simulink model "autopilot"  (R2016a)
settings: Solver=VariableStepAuto  StartTime=0.0  StopTime=inf  FixedStep=0.05  RelTol=1e-3
libraries: xpcutilitieslib x2, xpcobsoletelib x2, instrumentlib x2
settings Model: Creator=IEE12  LastModifiedBy=Marcelo
settings DataIOCC: LimitDataPoints=on  SaveFormat=Array
settings DebuggingCC: UnderspecifiedInitializationDetection=Classic  MergeDetectMultiDrivingBlocksExec=none  SolverPrmCheckMsg=warning  StateNameClashWarn=warning
settings HardwareCC: ProdBitPerPointer=32  ProdLargestAtomicFloat=None  ProdIntDivRoundTo=Undefined  ProdEndianess=Unspecified  ProdWordSize=32  ProdHWDeviceType=32-bit Generic
settings ModelReferenceCC: PropagateSignalLabelsOutOfModel=off
settings ConfigComp: CovModelRefEnable=Off

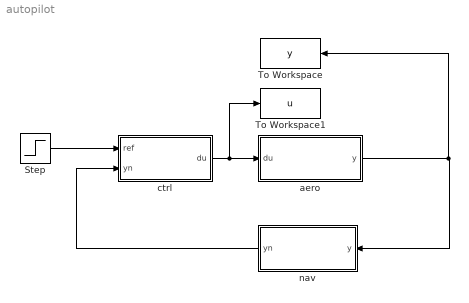
== system autopilot ==
  Step : Step  After=5  SampleTime=0
  To Workspace : ToWorkspace  VariableName=y  SaveFormat=Timeseries  SampleTime=-1
  To Workspace1 : ToWorkspace  VariableName=u  SaveFormat=Timeseries  SampleTime=-1
  aero : Subsystem
  ctrl : Subsystem
  nav : Subsystem
  wires:
  nav/1(yn) -> ctrl/2(yn)
  Step/1 -> ctrl/1(ref)
  ctrl/1(du) -> To Workspace1/1, aero/1(du)
  aero/1("y ") -> To Workspace/1, nav/1(y)

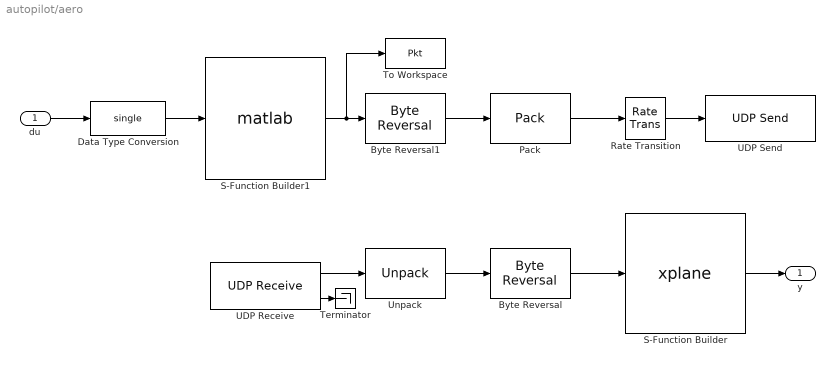
== system autopilot/aero ==
  du : Inport
  Byte Reversal : xpcutilitieslib/Byte Reversal   numInp=1
  Byte Reversal1 : xpcutilitieslib/Byte Reversal   numInp=1
  Data Type Conversion : DataTypeConversion  OutDataTypeStr=single
  Pack : xpcobsoletelib/Utilities/Pack   datatypes={'uint8'}  byteAlign=1
  Rate Transition : RateTransition  OutPortSampleTime=0.05
  S-Function Builder : S-Function  InitFcn=try, set_param(gcb,'FunctionName','xplane'), end  FunctionName=xplane  SFunctionModules=xplane_wrapper  SFunctionDeploymentMode=off  EnableBusSupport=off  mask(S-Function Builder){}
      mask help: Simulink:masks:SFunctionBuilder_MD
      mask init:
      | val = [[.9  0.75 0.75 1 1 .9 .9 1]',[1 1 0.75 0.75 .9 .9 1 .9]'];try , sys = get_param(gcb,'SfunBuilderFcnName');if isempty(sys), sys = get_param(gcb,'FunctionName'); end,catch, sys = get_param(gcb,'FunctionName'); end
      settings: CopyFcn=set_param(gcbh,'LinkStatus','none')  PreSaveFcn=try, set_param(gcb,'FunctionName','xplane'), end  OpenFcn=sfunctionwizard(gcbh)
      mask Display: plot(val(:,1),val(:,2)),disp(sys), port_label('input',1,'Pkt'), port_label('output',1,'y')
  S-Function Builder1 : S-Function  InitFcn=try, set_param(gcb,'FunctionName','matlab'), end  FunctionName=matlab  SFunctionModules=matlab_wrapper  SFunctionDeploymentMode=off  EnableBusSupport=off  mask(S-Function Builder){}
      mask help: Simulink:masks:SFunctionBuilder_MD
      mask init: same as autopilot/aero/S-Function Builder
      settings: CopyFcn=set_param(gcbh,'LinkStatus','none')  PreSaveFcn=try, set_param(gcb,'FunctionName','matlab'), end  OpenFcn=sfunctionwizard(gcbh)
      mask Display: plot(val(:,1),val(:,2)),disp(sys), port_label('input',1,'du'), port_label('output',1,'Pkt')
  Terminator : Terminator
  To Workspace : ToWorkspace  VariableName=Pkt  SaveFormat=Timeseries  SampleTime=-1
  UDP Receive : instrumentlib/UDP Receive  Host=127.0.0.1  Port=49001  LocalPort=49004  DataSize=257  EnableBlockingMode=off  Timeout=10  SampleTime=0.05  DataType=uint8  ByteOrder=BigEndian
  UDP Send : instrumentlib/UDP Send  Host=127.0.0.1  Port=49000  LocalPort=-1  EnableBlockingMode=on  ByteOrder=BigEndian
  Unpack : xpcobsoletelib/Utilities/Unpack   dimensions={[1 257]}  datatypes={'uint8'}  byteAlign=1
  "y " : Outport
  wires:
  UDP Receive/2 -> Terminator/1
  UDP Receive/1 -> Unpack/1
  Unpack/1 -> Byte Reversal/1
  Byte Reversal1/1 -> Pack/1
  S-Function Builder1/1 -> To Workspace/1, Byte Reversal1/1
  Data Type Conversion/1 -> S-Function Builder1/1
  Pack/1 -> Rate Transition/1
  Rate Transition/1 -> UDP Send/1
  du/1 -> Data Type Conversion/1
  S-Function Builder/1 -> "y "/1
  Byte Reversal/1 -> S-Function Builder/1

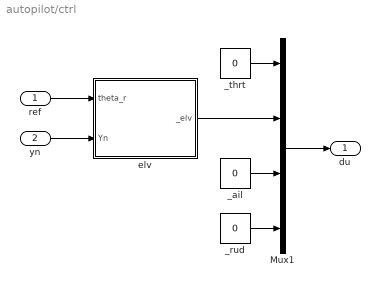
== system autopilot/ctrl ==
  ref : Inport
  yn : Inport  Port=2
  Mux1 : Mux
  _ail : Constant  Value=0
  _rud : Constant  Value=0
  _thrt : Constant  Value=0
  elv : Subsystem
  du : Outport
  wires:
  ref/1 -> elv/1(theta_r)
  yn/1 -> elv/2(Yn)
  Mux1/1 -> du/1
  _rud/1 -> Mux1/4
  _thrt/1 -> Mux1/1
  _ail/1 -> Mux1/3
  elv/1(_elv) -> Mux1/2

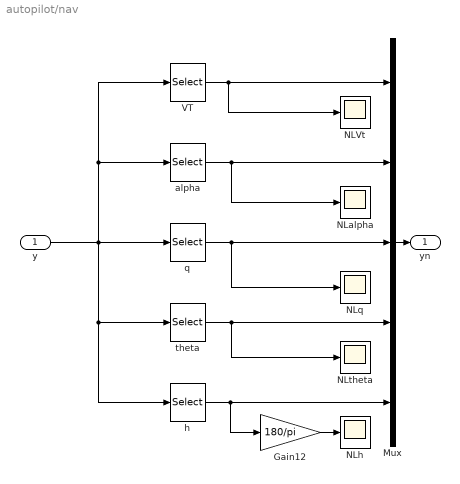
== system autopilot/nav ==
  y : Inport
  Gain12 : Gain  Gain=180/pi
  Mux : Mux  Inputs=5
  NLVt : Scope
  NLalpha : Scope
  NLh : Scope
  NLq : Scope
  NLtheta : Scope
  VT : Selector  InputPortWidth=12  IndexOptions=Index vector (dialog)  Indices=[1]  OutputSizes=1
  alpha : Selector  InputPortWidth=12  IndexOptions=Index vector (dialog)  Indices=[2]  OutputSizes=1
  h : Selector  InputPortWidth=12  IndexOptions=Index vector (dialog)  Indices=[12]  OutputSizes=1
  q : Selector  InputPortWidth=12  IndexOptions=Index vector (dialog)  Indices=[5]  OutputSizes=1
  theta : Selector  InputPortWidth=12  IndexOptions=Index vector (dialog)  Indices=[8]  OutputSizes=1
  yn : Outport
  wires:
  VT/1 -> NLVt/1, Mux/1
  y/1 -> VT/1, alpha/1, h/1, theta/1, q/1
  h/1 -> Gain12/1, Mux/5
  alpha/1 -> NLalpha/1, Mux/2
  q/1 -> NLq/1, Mux/3
  theta/1 -> NLtheta/1, Mux/4
  Mux/1 -> yn/1
  Gain12/1 -> NLh/1

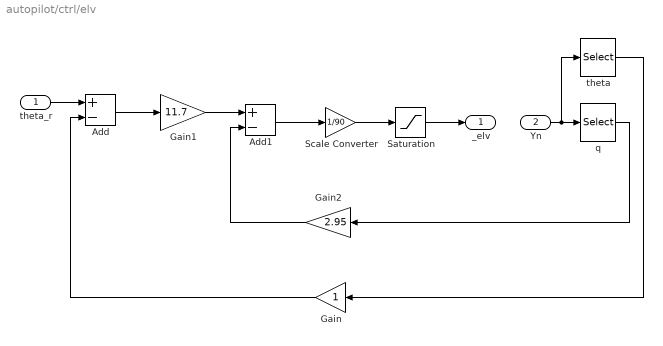
== system autopilot/ctrl/elv ==
  theta_r : Inport
  Yn : Inport  Port=2
  Add : Sum  Inputs=+-
  Add1 : Sum  Inputs=+-
  Gain : Gain
  Gain1 : Gain  Gain=11.7
  Gain2 : Gain  Gain=2.95
  Saturation : Saturate  UpperLimit=1.0  LowerLimit=-1.0
  Scale Converter : Gain  Gain=1/90
  q : Selector  InputPortWidth=5  IndexOptions=Index vector (dialog)  Indices=[3]  OutputSizes=1
  theta : Selector  InputPortWidth=5  IndexOptions=Index vector (dialog)  Indices=[4]  OutputSizes=1
  _elv : Outport
  wires:
  theta/1 -> Gain/1
  q/1 -> Gain2/1
  Add/1 -> Gain1/1
  Scale Converter/1 -> Saturation/1
  theta_r/1 -> Add/1
  Gain/1 -> Add/2
  Gain1/1 -> Add1/1
  Gain2/1 -> Add1/2
  Add1/1 -> Scale Converter/1
  Saturation/1 -> _elv/1
  Yn/1 -> theta/1, q/1
